simulink model "sixth"  (R2018a)
settings: Solver=VariableStepAuto  StartTime=0.0  StopTime=10.0  RelTol=1e-3
values from neighbouring files (symbols this model uses):
  kd = 0.2    [matlab.mat]
  ki = 0.01    [matlab.mat]
  kp = 0.2    [matlab.mat]
  Qs = 0.125    [matlab.mat]
  R = 1.6    [matlab.mat]
settings Model: Creator=Master  LastModifiedBy=Master

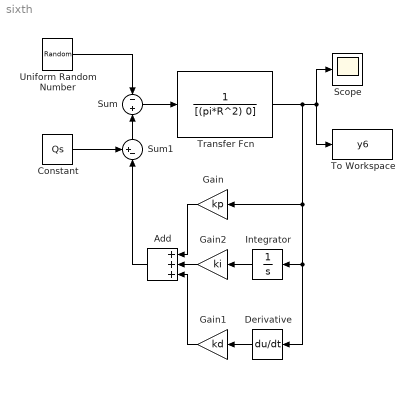
== system sixth ==
  Add : Sum  Inputs=+++
  Constant : Constant  Value=Qs
  Derivative : Derivative
  Gain : Gain  Gain=kp
  Gain1 : Gain  Gain=kd
  Gain2 : Gain  Gain=ki
  Integrator : Integrator
  Scope : Scope
  Sum : Sum  Inputs=-|+
  Sum1 : Sum  Inputs=+-|
  To Workspace : ToWorkspace  VariableName=y6  SaveFormat=Timeseries  SampleTime=-1
  Transfer Fcn : TransferFcn  Denominator=[(pi*R^2) 0]
  Uniform Random Number : UniformRandomNumber  SampleTime=0.1
  wires:
  Uniform Random Number/1 -> Sum/1
  Constant/1 -> Sum1/1
  Sum/1 -> Transfer Fcn/1
  Transfer Fcn/1 -> To Workspace/1, Scope/1, Derivative/1, Integrator/1, Gain/1
  Sum1/1 -> Sum/2
  Gain2/1 -> Add/2
  Integrator/1 -> Gain2/1
  Add/1 -> Sum1/2
  Derivative/1 -> Gain1/1
  Gain1/1 -> Add/3
  Gain/1 -> Add/1
